simulink model "Ex4_10"  (Simulink 6.0)
settings: Solver=FixedStepDiscrete  StartTime=0.0  StopTime=Tstop  RelTol=1e-3
values from neighbouring files (symbols this model uses):
  GAIN1 = 2    [Ex4_10_launch.m]
  GAIN2 = 2    [Ex4_10_launch.m]
  GAIN3 = 2    [Ex4_10_launch.m]
  initial = -1    [Ex4_10_launch.m]
  slope = 2/Tstop    (= 0.000100502512563)    [Ex4_10_launch.m]
  V_DAC_H = 0.5    [Ex4_10_launch.m]
  V_DAC_L = -0.5    [Ex4_10_launch.m]
  VthH1 = 0.18    [Ex4_10_launch.m]
  VthH2 = 0.19    [Ex4_10_launch.m]
  VthH3 = 0.25    [Ex4_10_launch.m]
  VthL1 = -0.25    [Ex4_10_launch.m]
  VthL2 = -0.28    [Ex4_10_launch.m]
  VthL3 = -0.25    [Ex4_10_launch.m]
libraries: simulink x1
settings Model: Creator=francomaloberti  LastModifiedBy=Cri  ExtModeAutoUpdateStatusClock=off
settings DataIOCC: SignalLoggingName=sigsOut
settings OptimizationCC: InlineInvariantSignals=off
settings DebuggingCC: SolverPrmCheckMsg=none
settings HardwareCC: TargetUnknown=on

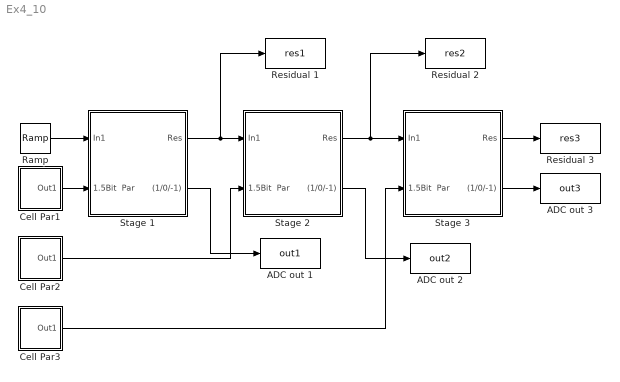
== system Ex4_10 ==
  ADC out 1 : ToWorkspace  VariableName=out1  SampleTime=-1  SaveFormat=Array
  ADC out 2 : ToWorkspace  VariableName=out2  SampleTime=-1  SaveFormat=Array
  ADC out 3 : ToWorkspace  VariableName=out3  SampleTime=-1  SaveFormat=Array
  Cell Par1 : Subsystem
  Cell Par2 : Subsystem
  Cell Par3 : Subsystem
  Ramp : simulink/Sources/Ramp  slope=slope  start=0  X0=initial
  Residual 1 : ToWorkspace  VariableName=res1  SampleTime=-1  SaveFormat=Array
  Residual 2 : ToWorkspace  VariableName=res2  SampleTime=-1  SaveFormat=Array
  Residual 3 : ToWorkspace  VariableName=res3  SampleTime=-1  SaveFormat=Array
  Stage 1 : Subsystem
  Stage 2 : Subsystem
  Stage 3 : Subsystem
  wires:
  Cell Par1/1(Out1) -> Stage 1/2(1.5Bit  Par)
  Ramp/1 -> Stage 1/1(In1)
  Stage 1/1(Res) -> Residual 1/1, Stage 2/1(In1)
  Stage 1/2((1/0/-1)) -> ADC out 1/1
  Stage 2/2((1/0/-1)) -> ADC out 2/1
  Stage 2/1(Res) -> Residual 2/1, Stage 3/1(In1)
  Stage 3/2((1/0/-1)) -> ADC out 3/1
  Cell Par2/1(Out1) -> Stage 2/2(1.5Bit  Par)
  Stage 3/1(Res) -> Residual 3/1
  Cell Par3/1(Out1) -> Stage 3/2(1.5Bit  Par)

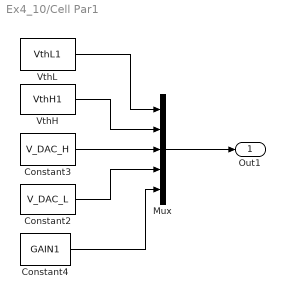
== system Ex4_10/Cell Par1 ==
  Constant2 : Constant  Value=V_DAC_L
  Constant3 : Constant  Value=V_DAC_H
  Constant4 : Constant  Value=GAIN1
  Mux : Mux  Inputs=5
  VthH : Constant  Value=VthH1
  VthL : Constant  Value=VthL1
  Out1 : Outport
  wires:
  Mux/1 -> Out1/1
  VthL/1 -> Mux/1
  VthH/1 -> Mux/2
  Constant4/1 -> Mux/5
  Constant3/1 -> Mux/3
  Constant2/1 -> Mux/4

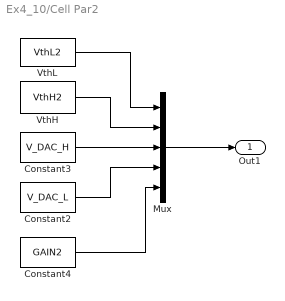
== system Ex4_10/Cell Par2 ==
  Constant2 : Constant  Value=V_DAC_L
  Constant3 : Constant  Value=V_DAC_H
  Constant4 : Constant  Value=GAIN2
  Mux : Mux  Inputs=5
  VthH : Constant  Value=VthH2
  VthL : Constant  Value=VthL2
  Out1 : Outport
  wires:
  Constant2/1 -> Mux/4
  Constant3/1 -> Mux/3
  Constant4/1 -> Mux/5
  VthH/1 -> Mux/2
  VthL/1 -> Mux/1
  Mux/1 -> Out1/1

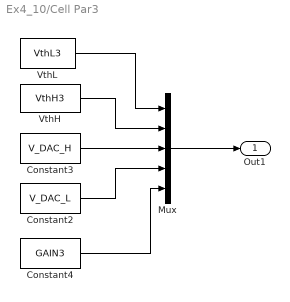
== system Ex4_10/Cell Par3 ==
  Constant2 : Constant  Value=V_DAC_L
  Constant3 : Constant  Value=V_DAC_H
  Constant4 : Constant  Value=GAIN3
  Mux : Mux  Inputs=5
  VthH : Constant  Value=VthH3
  VthL : Constant  Value=VthL3
  Out1 : Outport
  wires:
  Mux/1 -> Out1/1
  VthL/1 -> Mux/1
  VthH/1 -> Mux/2
  Constant4/1 -> Mux/5
  Constant3/1 -> Mux/3
  Constant2/1 -> Mux/4

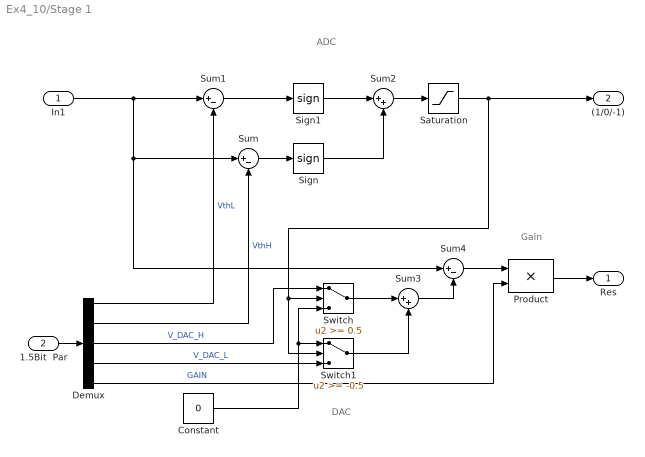
== system Ex4_10/Stage 1 ==
  note: Gain
  note: DAC
  note: ADC
  In1 : Inport  Port=1  LatchInput=off
  1.5Bit  Par : Inport  Port=2  LatchInput=off
  Constant : Constant  Value=0
  Demux : Demux  Outputs=5
  Product : Product  SaturateOnIntegerOverflow=on
  Saturation : Saturate  UpperLimit=1  LowerLimit=-1
  Sign : Signum
  Sign1 : Signum
  Sum : Sum  Inputs=|+-  SaturateOnIntegerOverflow=on
  Sum1 : Sum  Inputs=|+-  SaturateOnIntegerOverflow=on
  Sum2 : Sum  Inputs=|++  SaturateOnIntegerOverflow=on
  Sum3 : Sum  Inputs=|++  SaturateOnIntegerOverflow=on
  Sum4 : Sum  Inputs=|+-  SaturateOnIntegerOverflow=on
  Switch : Switch  Threshold=0.5  SaturateOnIntegerOverflow=on
  Switch1 : Switch  Threshold=-0.5  SaturateOnIntegerOverflow=on
  Res : Outport
  (1/0/-1) : Outport  Port=2
  wires:
  Sum4/1 -> Product/1
  Sum3/1 -> Sum4/2
  Product/1 -> Res/1
  Demux/5 -> Product/2  "GAIN"
  Constant/1 -> Switch1/1, Switch/3
  Demux/4 -> Switch1/3  "V_DAC_L"
  Switch1/1 -> Sum3/2
  Switch/1 -> Sum3/1
  Demux/3 -> Switch/1  "V_DAC_H"
  Saturation/1 -> (1/0/-1)/1, Switch/2, Switch1/2
  Sum2/1 -> Saturation/1
  Sign/1 -> Sum2/2
  Sign1/1 -> Sum2/1
  In1/1 -> Sum4/1, Sum/1, Sum1/1
  Demux/2 -> Sum/2  "VthH"
  Demux/1 -> Sum1/2  "VthL"
  Sum1/1 -> Sign1/1
  Sum/1 -> Sign/1
  1.5Bit  Par/1 -> Demux/1

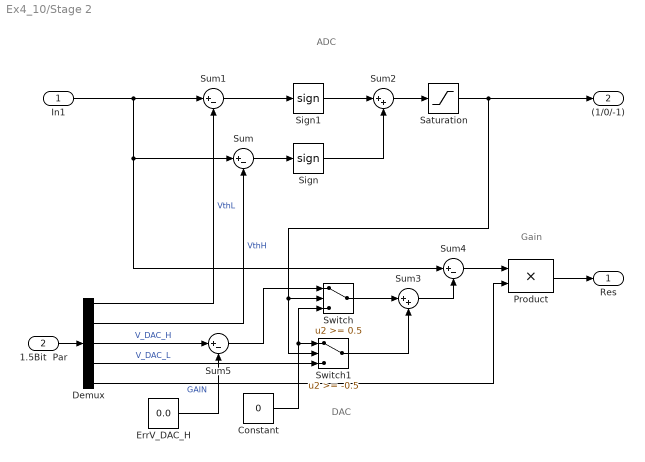
== system Ex4_10/Stage 2 ==
  note: ADC
  note: DAC
  note: Gain
  In1 : Inport  Port=1  LatchInput=off
  1.5Bit  Par : Inport  Port=2  LatchInput=off
  Constant : Constant  Value=0
  Demux : Demux  Outputs=5
  ErrV_DAC_H : Constant  Value=0.0
  Product : Product  SaturateOnIntegerOverflow=on
  Saturation : Saturate  UpperLimit=1  LowerLimit=-1
  Sign : Signum
  Sign1 : Signum
  Sum{,1,4..5} (4 alike) : Sum  Inputs=|+-  SaturateOnIntegerOverflow=on
  Sum2 : Sum  Inputs=|++  SaturateOnIntegerOverflow=on
  Sum3 : Sum  Inputs=|++  SaturateOnIntegerOverflow=on
  Switch : Switch  Threshold=0.5  SaturateOnIntegerOverflow=on
  Switch1 : Switch  Threshold=-0.5  SaturateOnIntegerOverflow=on
  Res : Outport
  (1/0/-1) : Outport  Port=2
  wires:
  1.5Bit  Par/1 -> Demux/1
  Sum/1 -> Sign/1
  Sum1/1 -> Sign1/1
  Demux/1 -> Sum1/2  "VthL"
  Demux/2 -> Sum/2  "VthH"
  In1/1 -> Sum1/1, Sum4/1, Sum/1
  Sign1/1 -> Sum2/1
  Sign/1 -> Sum2/2
  Sum2/1 -> Saturation/1
  Saturation/1 -> Switch1/2, Switch/2, (1/0/-1)/1
  Switch/1 -> Sum3/1
  Switch1/1 -> Sum3/2
  Demux/4 -> Switch1/3  "V_DAC_L"
  Constant/1 -> Switch/3, Switch1/1
  Demux/5 -> Product/2  "GAIN"
  Product/1 -> Res/1
  Sum3/1 -> Sum4/2
  Sum4/1 -> Product/1
  Demux/3 -> Sum5/1  "V_DAC_H"
  Sum5/1 -> Switch/1
  ErrV_DAC_H/1 -> Sum5/2

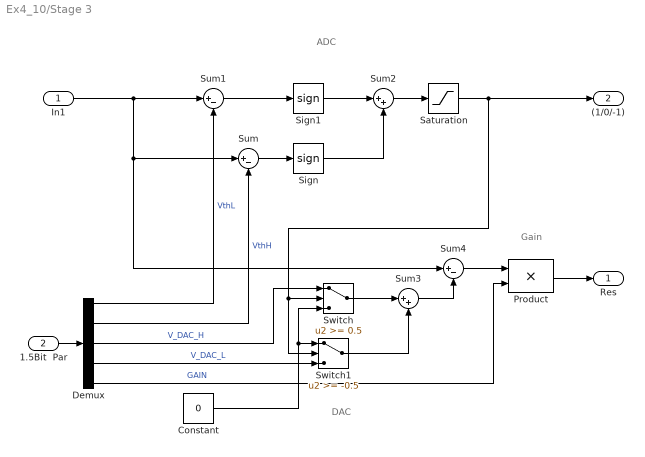
== system Ex4_10/Stage 3 ==
  note: ADC
  note: DAC
  note: Gain
  In1 : Inport  Port=1  LatchInput=off
  1.5Bit  Par : Inport  Port=2  LatchInput=off
  Constant : Constant  Value=0
  Demux : Demux  Outputs=5
  Product : Product  SaturateOnIntegerOverflow=on
  Saturation : Saturate  UpperLimit=1  LowerLimit=-1
  Sign : Signum
  Sign1 : Signum
  Sum : Sum  Inputs=|+-  SaturateOnIntegerOverflow=on
  Sum1 : Sum  Inputs=|+-  SaturateOnIntegerOverflow=on
  Sum2 : Sum  Inputs=|++  SaturateOnIntegerOverflow=on
  Sum3 : Sum  Inputs=|++  SaturateOnIntegerOverflow=on
  Sum4 : Sum  Inputs=|+-  SaturateOnIntegerOverflow=on
  Switch : Switch  Threshold=0.5  SaturateOnIntegerOverflow=on
  Switch1 : Switch  Threshold=-0.5  SaturateOnIntegerOverflow=on
  Res : Outport
  (1/0/-1) : Outport  Port=2
  wires:
  1.5Bit  Par/1 -> Demux/1
  Sum/1 -> Sign/1
  Sum1/1 -> Sign1/1
  Demux/1 -> Sum1/2  "VthL"
  Demux/2 -> Sum/2  "VthH"
  In1/1 -> Sum1/1, Sum/1, Sum4/1
  Sign1/1 -> Sum2/1
  Sign/1 -> Sum2/2
  Sum2/1 -> Saturation/1
  Saturation/1 -> Switch1/2, Switch/2, (1/0/-1)/1
  Demux/3 -> Switch/1  "V_DAC_H"
  Switch/1 -> Sum3/1
  Switch1/1 -> Sum3/2
  Demux/4 -> Switch1/3  "V_DAC_L"
  Constant/1 -> Switch/3, Switch1/1
  Demux/5 -> Product/2  "GAIN"
  Product/1 -> Res/1
  Sum3/1 -> Sum4/2
  Sum4/1 -> Product/1
